simulink model "WindTurbineSystem"  (R2023b)
settings: Solver=VariableStepAuto  StartTime=0.0  StopTime=simT  RelTol=1e-3
settings Model: Creator=FRESH  LastModifiedBy=FRESH
settings SimscapeCC: SimscapeLogSimulationStatistics=on

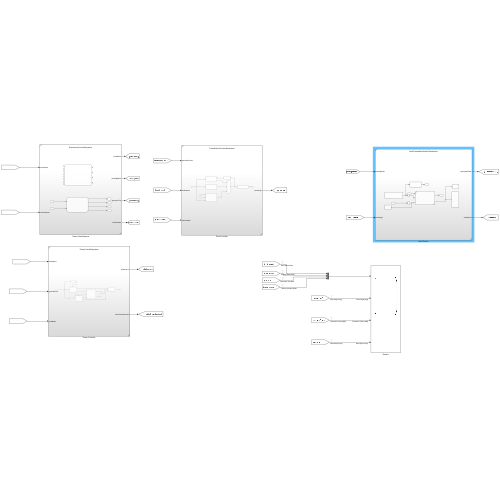
[thumbnail: Simulink's stored preview of the top-level diagram]
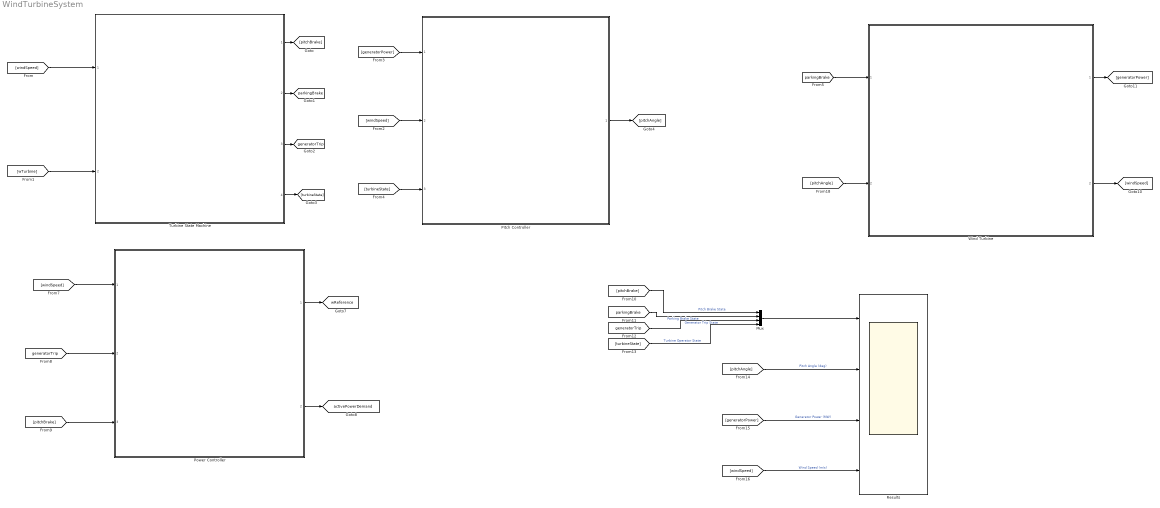
== system WindTurbineSystem ==
  Mux : Mux
  Pitch Controller : Subsystem  ReferencedSubsystem=TurbinePitchControllerSubsystem
  Power Controller : Subsystem  ReferencedSubsystem=PowerControlSubsystem
  Results : Scope  NumInputPorts=4
  Turbine State Machine : Subsystem  ReferencedSubsystem=SupervisoryControlSubsystem
  Wind Turbine : Subsystem  ReferencedSubsystem=WindTurbineWithGridAndTransformer
  tag scope: activePowerDemand=global, generatorTrip=global, parkingBrake=global, wReference=global
  wires:
  Mux/1 -> Results/1
  [windSpeed] -> Turbine State Machine/1
  [wTurbine] -> Turbine State Machine/2
  Turbine State Machine/1 -> [pitchBrake]
  Turbine State Machine/2 -> [parkingBrake]
  Turbine State Machine/3 -> [generatorTrip]
  Turbine State Machine/4 -> [turbineState]
  Power Controller/1 -> [wReference]
  Power Controller/2 -> [activePowerDemand]
  [windSpeed] -> Power Controller/1
  [generatorTrip] -> Power Controller/2
  [pitchBrake] -> Power Controller/3
  [pitchBrake] -> Mux/1  "Pitch Brake State"
  [parkingBrake] -> Mux/2  "Parking Brake State"
  [generatorTrip] -> Mux/3  "Generator Trip State"
  [turbineState] -> Mux/4  "Turbine Operator State"
  [pitchAngle] -> Results/2  "Pitch Angle (deg)"
  [generatorPower] -> Results/3  "Generator Power (MW)"
  [windSpeed] -> Results/4  "Wind Speed (m/s)"
  [windSpeed] -> Pitch Controller/2
  [generatorPower] -> Pitch Controller/1
  [turbineState] -> Pitch Controller/3
  Pitch Controller/1 -> [pitchAngle]
  Wind Turbine/1 -> [generatorPower]
  [pitchAngle] -> Wind Turbine/2
  Wind Turbine/2 -> [windSpeed]
  [parkingBrake] -> Wind Turbine/1
